simulink model "BLDCmotorControl_FOC_R2017b"  (R2017b)
settings: Solver=FixedStepDiscrete  StartTime=0  StopTime=1  FixedStep=Ts  MaxStep=1e-6  RelTol=1e-6  AbsTol=1e-6  EnableMultiTasking=on
PreLoadFcn:
  | addpath(genpath('01_Libraries'));
  | addpath(genpath('02_Figures'));
InitFcn:
  | init_model;
values from neighbouring files (symbols this model uses):
  a_elecAngle = 60    [init_model_Ffwd.m]
  a_elecPeriod = 360    [init_model_Ffwd.m]
  b_DCLinkCurrAvail = 0    [init_model_Ffwd.m]
  b_selPhaABCurrMeas = 1    [init_model_Ffwd.m]
  cf_speedCoef = round(f_ctrl * a_mechAngle * (pi/180) * (30/pi))    [init_model_Ffwd.m]
  i_thresOutlier = 200    [init_model_Ffwd.m]
  n_commAcvLo = 15    [init_model_Ffwd.m]
  n_commDeacvHi = 30    [init_model_Ffwd.m]
  r_sin_M1 = sin((a_elecAngle_XA + 30)*(pi/180))    [init_model_Ffwd.m]
  r_whl = 6.5 * 2.54 * 1e-2 / 2    (= 0.08255)    [init_model_Ffwd.m]
  res_elecAngle = 2    [init_model_Ffwd.m]
  Ts = 5e-6    (= 5e-06)    [init_model_Ffwd.m]    (also in pe_electric_engine_dyno_data.m = 1e-05)
  Ts_ctrl = 6e-5    (= 6e-05)    [init_model_Ffwd.m]
  vec_hallToPos = [0 2 0 1 4 3 5 0]    [init_model_Ffwd.m]
  z_commutMap_M1 = [-1 -1  0  1  1  0 ... (first row only)    [init_model_Ffwd.m]
  z_ctrlTypSel = 1    [init_model_Ffwd.m]
  z_maxCntRst = 2000    [init_model_Ffwd.m]
undefined symbols (not defined in the file or in its folder): a_phaAdv_M1, b_phaAdvEna, CTRL_COMM, DiscIntNeverNeededParam, Down, dz_counterHi, dz_counterLo, Kb_Id, Kb_Iq, Kb_n, Ki_Id, Ki_Iq, Ki_n, Kp_Id, Kp_Iq, Kp_n, n_motPhaAdvEna, r_commDCDeacv, sigbuilder_block, Up, V_circleLim_M1, V_max, V_min
libraries: pePwmGenerator x7, BLDC_controller_Lib x6, powerlib x6, simulink x5
(part 1 of 3)
Description:
  | This example illustrates use of the BLDC in a closed-loop
  | speed and voltage control on a 1 kW, 3000 rpm industrial motor
  | 
  | 
  | Copyright 2008-2019 The MathWorks, Inc.
settings Model: ExtModeAutoUpdateStatusClock=off  TunableVars=Ki_Id,Ki_Iq,Kp_Id,Kp_Iq,a_phaAdv_M1,b_phaAdvEna,cf_speedCoef,cf_speedFilt,dz_counterHi,dz_counterLo,f_ctrl,n_commAcvLo,n_commDeacvHi,n_motPhaAdvEna,r_commDCDeacv,r_phaAdvDC_XA,z_ctrlTypSel,z_maxCntRst  TunableVarsStorageClass=Auto,Auto,Auto,Auto,Auto,Auto,Auto,Auto,Auto,Auto,Auto,Auto,Auto,Auto,Auto,Auto,Auto,Auto  TunableVarsTypeQualifier=,,,,,,,,,,,,,,,,,  Creator=MathWorks  LastModifiedBy=37ef
settings SolverCC: AutoInsertRateTranBlk=on
settings DataIOCC: LimitDataPoints=on  SaveFormat=Array  ReturnWorkspaceOutputs=on  SignalLoggingName=sigsOut
settings OptimizationCC: DefaultParameterBehavior=Inlined  UseDivisionForNetSlopeComputation=on  UseFloatMulNetSlope=on  UseSpecifiedMinMax=on  InlineInvariantSignals=on  PassReuseOutputArgsAs=Individual arguments  ExpressionDepthLimit=2147483647  ZeroExternalMemoryAtStartup=off  ZeroInternalMemoryAtStartup=off  NoFixptDivByZeroProtection=on  EfficientFloat2IntCast=on  LifeSpan=1  OptimizeBlockOrder=speed  DifferentSizesBufferReuse=on
settings DebuggingCC: ReadBeforeWriteMsg=DisableAll  WriteAfterWriteMsg=DisableAll  WriteAfterReadMsg=DisableAll  UnderspecifiedInitializationDetection=Classic  InheritedTsInSrcMsg=none  MultiTaskDSMMsg=none  MultiTaskCondExecSysMsg=none  ParameterTunabilityLossMsg=error  FcnCallInpInsideContextMsg=warning  StateNameClashWarn=warning  SFUnexpectedBacktrackingDiag=warning  SFNoUnconditionalDefaultTransitionDiag=warning  SFExecutionAtInitializationDiag=none
settings HardwareCC: ProdBitPerPointer=32  ProdBitPerSizeT=32  ProdBitPerPtrDiffT=32  ProdLargestAtomicInteger=Long  ProdLargestAtomicFloat=Double  ProdWordSize=32  ProdHWDeviceType=ARM Compatible->ARM Cortex  TargetBitPerPointer=64  TargetBitPerSizeT=64  TargetBitPerPtrDiffT=64  TargetLongLongMode=on  TargetIntDivRoundTo=Zero  TargetEndianess=LittleEndian  TargetWordSize=64  TargetHWDeviceType=MATLAB Host  ProdEqTarget=off
settings ModelReferenceCC: UpdateModelReferenceTargets=IfOutOfDate  PropagateSignalLabelsOutOfModel=off
settings SFSimCC: SFSimEcho=off  MATLABDynamicMemAlloc=off
settings RTWCC: SystemTargetFile=ert.tlc  GenCodeOnly=on  TemplateMakefile=ert_default_tmf  GenerateReport=on  BuildConfiguration=Faster Runs  IncludeHyperlinkInReport=on  LaunchReport=on  GenerateTraceInfo=on  GenerateTraceReport=on  GenerateTraceReportSl=on  GenerateTraceReportSf=on  GenerateTraceReportEml=on  GenerateCodeMetricsReport=on  GenerateCodeReplacementReport=on
settings CodeAppCC: ForceParamTrailComments=on  IgnoreCustomStorageClasses=off  OperatorAnnotations=on  SimulinkDataObjDesc=on  SFDataObjDesc=on  CustomSymbolStrGlobalVar=rt$N$M  CustomSymbolStrType=$N$M  CustomSymbolStrFcn=$N$M$F  CustomSymbolStrMacro=$N$M  InsertBlockDesc=on
settings ERTTargetCC: GenerateSampleERTMain=on  IncludeMdlTerminateFcn=off  CombineSignalStateStructs=on  SuppressErrorStatus=on  MultiInstanceERTCode=on  CodeInterfacePackaging=Reusable function  SupportNonFinite=off  SupportComplex=off  InlinedParameterPlacement=NonHierarchical  RootIOFormat=Part of model data structure  ERTCustomFileTemplate=example_file_process.tlc  ERTFilePackagingFormat=CompactWithDataFile  PreserveStaticInFcnDecls=off
settings ConfigComp: CovMetricSettings=dw  CovHtmlReporting=on  CovSaveCumulativeToWorkspaceVar=on  CovSaveSingleToWorkspaceVar=on  CovExternalEMLEnable=off  CovSFcnEnable=off
settings SimscapeCC: SimscapeNormalizeSystem=off

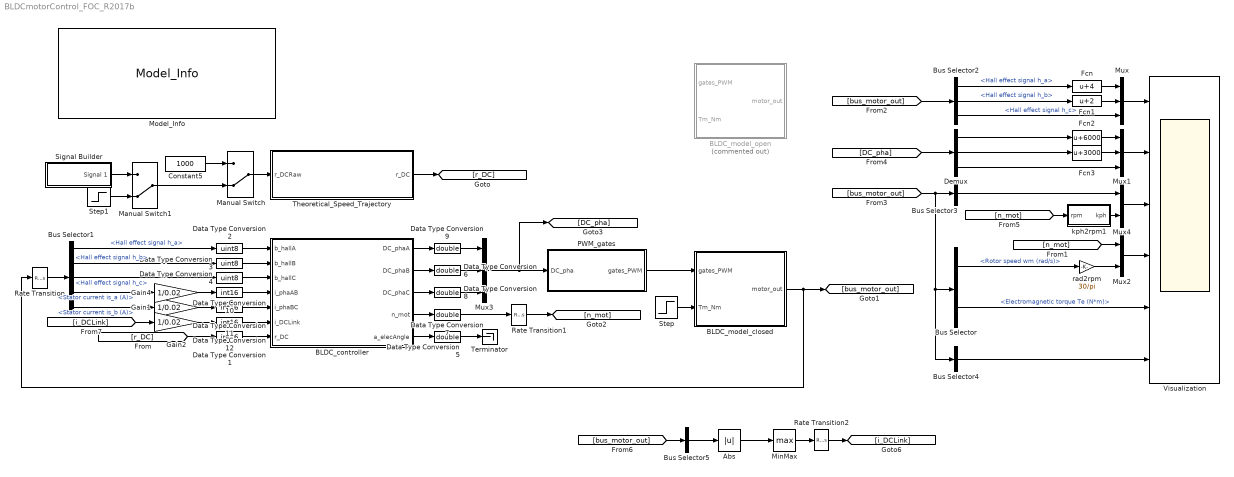
== system BLDCmotorControl_FOC_R2017b ==
  Abs : Abs
  BLDC_controller : Subsystem  TreatAsAtomicUnit=on  SystemSampleTime=Ts_ctrl
  BLDC_model_closed : Subsystem
      mask help: Simulink:masks:GenSFuncDesc_MD
      mask Help: eval('feval(''rtwprivate'',''rtwhelpview'',''rtw_sfcn_block'')');
  BLDC_model_open : Subsystem  Commented=on
  Bus Selector : BusSelector  OutputSignals=Rotor speed wm (rad/s),Electromagnetic torque Te (N*m)
  Bus Selector1 : BusSelector  OutputSignals=Hall effect signal h_a,Hall effect signal h_b,Hall effect signal h_c,Stator current is_a (A),Stator current is_b (A)
  Bus Selector2 : BusSelector  OutputSignals=Hall effect signal h_a,Hall effect signal h_b,Hall effect signal h_c
  Bus Selector3 : BusSelector  OutputSignals=Stator current is_a (A),Stator current is_b (A),Stator current is_c (A)  OutputAsBus=on
  Bus Selector4 : BusSelector  OutputSignals=Stator back EMF e_a (V),Stator back EMF e_b (V),Stator back EMF e_cV)  OutputAsBus=on
  Bus Selector5 : BusSelector  OutputSignals=Stator current is_a (A),Stator current is_b (A),Stator current is_c (A)  OutputAsBus=on
  Constant5 : Constant  Value=1000  OutDataTypeStr=double
  Data Type Conversion{1,10..12} (4 alike) : DataTypeConversion  OutDataTypeStr=int16  RndMeth=Zero
  Data Type Conversion2 : DataTypeConversion  OutDataTypeStr=uint8  RndMeth=Zero
  Data Type Conversion3 : DataTypeConversion  OutDataTypeStr=uint8  RndMeth=Zero
  Data Type Conversion4 : DataTypeConversion  OutDataTypeStr=uint8  RndMeth=Zero
  Data Type Conversion{5..9} (5 alike) : DataTypeConversion  OutDataTypeStr=double  RndMeth=Zero
  Demux : Demux  Outputs=3
  Fcn : Fcn  Expr=u+4
  Fcn1 : Fcn  Expr=u+2
  Fcn2 : Fcn  Expr=u+6000
  Fcn3 : Fcn  Expr=u+3000
  Gain1 : Gain  Tag=struct('comment',struct('text','','placement',1),'logdata',struct('maxnumvals',inf,'plotchannels',[],'loggingmode',3,'channels',1),'output',struct('variable','','description','','name','$S_$B','width',1,'address','','max',NaN,'min',NaN,'class','default','type','CONTINUOUS','scaling','','lsb',1,'offset',0,'arb',0,'freeze',1,'unit','','autoscalingmode',1,'lowerheadroom',1,'upperheadroom',1,'headroomunit','bit','keepdatatype',1,'checkmin',0,'checkmax',0,'castoutput',0,'show',0),'gain',struct('variable','','description','','name','$S_$B_gain','width',1,'address','','max',NaN,'min',NaN,'class','default','type','CONTINUOUS','scaling','','lsb',1,'offset',0,'arb',0,'freeze',1,'unit','','keepdatatype',1,'value','1','scalar',0,'tolerance',1),'scalingvalid',0,'date',730486)  Gain=1/0.02  RndMeth=Zero  SaturateOnIntegerOverflow=on  OutDataTypeStr=Inherit: Same as input  ParamDataTypeStr=Inherit: Same as input
  Gain2 : Gain  Tag=struct('comment',struct('text','','placement',1),'logdata',struct('maxnumvals',inf,'plotchannels',[],'loggingmode',3,'channels',1),'output',struct('variable','','description','','name','$S_$B','width',1,'address','','max',NaN,'min',NaN,'class','default','type','CONTINUOUS','scaling','','lsb',1,'offset',0,'arb',0,'freeze',1,'unit','','autoscalingmode',1,'lowerheadroom',1,'upperheadroom',1,'headroomunit','bit','keepdatatype',1,'checkmin',0,'checkmax',0,'castoutput',0,'show',0),'gain',struct('variable','','description','','name','$S_$B_gain','width',1,'address','','max',NaN,'min',NaN,'class','default','type','CONTINUOUS','scaling','','lsb',1,'offset',0,'arb',0,'freeze',1,'unit','','keepdatatype',1,'value','1','scalar',0,'tolerance',1),'scalingvalid',0,'date',730486)  Gain=1/0.02  RndMeth=Zero  SaturateOnIntegerOverflow=on  OutDataTypeStr=Inherit: Same as input  ParamDataTypeStr=Inherit: Same as input
  Gain4 : Gain  Tag=struct('comment',struct('text','','placement',1),'logdata',struct('maxnumvals',inf,'plotchannels',[],'loggingmode',3,'channels',1),'output',struct('variable','','description','','name','$S_$B','width',1,'address','','max',NaN,'min',NaN,'class','default','type','CONTINUOUS','scaling','','lsb',1,'offset',0,'arb',0,'freeze',1,'unit','','autoscalingmode',1,'lowerheadroom',1,'upperheadroom',1,'headroomunit','bit','keepdatatype',1,'checkmin',0,'checkmax',0,'castoutput',0,'show',0),'gain',struct('variable','','description','','name','$S_$B_gain','width',1,'address','','max',NaN,'min',NaN,'class','default','type','CONTINUOUS','scaling','','lsb',1,'offset',0,'arb',0,'freeze',1,'unit','','keepdatatype',1,'value','1','scalar',0,'tolerance',1),'scalingvalid',0,'date',730486)  Gain=1/0.02  RndMeth=Zero  SaturateOnIntegerOverflow=on  OutDataTypeStr=Inherit: Same as input  ParamDataTypeStr=Inherit: Same as input
  Manual Switch : ManualSwitch  CurrentSetting=0
  Manual Switch1 : ManualSwitch  CurrentSetting=0
  MinMax : MinMax  Function=max
  Model_Info : BLDC_controller_Lib/Model_Info
  Mux : Mux  Inputs=3
  Mux1 : Mux  Inputs=3
  Mux2 : Mux  Inputs=2
  Mux3 : Mux  Inputs=3
  Mux4 : Mux  Inputs=2
  PWM_gates : Subsystem
  Rate Transition : RateTransition  Integrity=off  Deterministic=off
  Rate Transition1 : RateTransition  Integrity=off  Deterministic=off
  Rate Transition2 : RateTransition  Integrity=off  Deterministic=off
  Signal Builder : Subsystem  Tag=STV Subsys  LoadFcn=sigbuilder_block('load');  StartFcn=sigbuilder_block('start');  StopFcn=sigbuilder_block('stop');  ClipboardFcn=sigbuilder_block('clipboard');  mask(Sigbuilder block){tuvar=[0:10]}
      mask help: Simulink:masks:SigbuilderBlock_MD
      mask init:
      | if ~strcmp(get_param(bdroot(gcbh),'SimulationStatus'),'stopped') tuvar = sigbuilder_block('maskInit'); end
      settings: CopyFcn=sigbuilder_block('copy');  DeleteFcn=sigbuilder_block('delete');  ModelCloseFcn=sigbuilder_block('modelClose');  PreSaveFcn=sigbuilder_block('preSave');  PauseFcn=sigbuilder_block('pause');  ContinueFcn=sigbuilder_block('continue');  NameChangeFcn=sigbuilder_block('namechange');  OpenFcn=sigbuilder_block('open',[141.283 165.057 550.868 400.075 ]);  CloseFcn=sigbuilder_block('close');
      mask Display: plot(0, 0, 100, 100,[2, 2, 32, 32, 2], [68, 8, 8, 68, 68],[32, 2], [38, 38], [32, 19, 2],[53, 60, 44], [32, 17, 17, 2],[16, 16, 31, 31]);txt = getActiveGroup(gcbh);text(2, 100, txt,'verticalAlignment', 'top');
  Step : Step  Time=0  After=0.5  SampleTime=0
  Step1 : Step  Time=0.25  Before=1000  After=-1000
  Terminator : Terminator
      settings: Tag=Controls_Lib  Description=Terminator  CopyFcn=Lib_CopyFcn(gcb);  PreDeleteFcn=Lib_PreDeleteFcn(gcb);
  Theoretical_Speed_Trajectory : Subsystem
  Visualization : Scope  NumInputPorts=6
  kph2rpm1 : Subsystem
  rad2rpm : Gain  Gain=30/pi
  wires:
  Mux2/1 -> Visualization/4
  Bus Selector/1 -> rad2rpm/1  "<Rotor speed wm (rad/s)>"
  Bus Selector/2 -> Visualization/5  "<Electromagnetic torque Te (N*m)>"
  Bus Selector2/3 -> Mux/3  "<Hall effect signal h_c>"
  Bus Selector2/2 -> Fcn1/1  "<Hall effect signal h_b>"
  Bus Selector2/1 -> Fcn/1  "<Hall effect signal h_a>"
  Fcn1/1 -> Mux/2
  Mux/1 -> Visualization/1
  Fcn/1 -> Mux/1
  Demux/1 -> Fcn2/1
  Demux/2 -> Fcn3/1
  Fcn2/1 -> Mux1/1
  Fcn3/1 -> Mux1/2
  Demux/3 -> Mux1/3
  Mux1/1 -> Visualization/2
  Bus Selector4/1 -> Visualization/6
  rad2rpm/1 -> Mux2/2
  BLDC_controller/4(n_mot) -> Data Type Conversion7/1
  BLDC_model_closed/1(motor_out) -> Rate Transition/1, [bus_motor_out]
  Step/1 -> BLDC_model_closed/2(Tm_Nm)
  Bus Selector1/2 -> Data Type Conversion3/1  "<Hall effect signal h_b>"
  Bus Selector1/1 -> Data Type Conversion2/1  "<Hall effect signal h_a>"
  Bus Selector1/3 -> Data Type Conversion4/1  "<Hall effect signal h_c>"
  Rate Transition/1 -> Bus Selector1/1
  Data Type Conversion2/1 -> BLDC_controller/1("b_hallA ")
  Data Type Conversion3/1 -> BLDC_controller/2(b_hallB)
  Data Type Conversion4/1 -> BLDC_controller/3(b_hallC)
  Theoretical_Speed_Trajectory/1(r_DC) -> [r_DC]
  [r_DC] -> Data Type Conversion1/1
  Data Type Conversion1/1 -> BLDC_controller/7(r_DC)
  BLDC_controller/2(DC_phaB) -> Data Type Conversion6/1
  BLDC_controller/3(DC_phaC) -> Data Type Conversion8/1
  BLDC_controller/1(DC_phaA) -> Data Type Conversion9/1
  Data Type Conversion7/1 -> Rate Transition1/1
  BLDC_controller/5(a_elecAngle) -> Data Type Conversion5/1
  Mux3/1 -> [DC_pha], PWM_gates/1(DC_pha)
  PWM_gates/1(gates_PWM) -> BLDC_model_closed/1(gates_PWM)
  Rate Transition1/1 -> [n_mot]
  [n_mot] -> Mux2/1
  [bus_motor_out] -> Bus Selector2/1
  [bus_motor_out] -> Bus Selector3/1, Bus Selector4/1, Bus Selector/1
  [DC_pha] -> Demux/1
  Manual Switch/1 -> Theoretical_Speed_Trajectory/1(r_DCRaw)
  Constant5/1 -> Manual Switch/1
  Signal Builder/1(Signal 1) -> Manual Switch1/1
  Manual Switch1/1 -> Manual Switch/2
  Step1/1 -> Manual Switch1/2
  Data Type Conversion5/1 -> Terminator/1
  Data Type Conversion8/1 -> Mux3/3
  Data Type Conversion6/1 -> Mux3/2
  Data Type Conversion9/1 -> Mux3/1
  [n_mot] -> kph2rpm1/1(rpm)
  Mux4/1 -> Visualization/3
  Bus Selector3/1 -> Mux4/1
  kph2rpm1/1(kph) -> Mux4/2
  Data Type Conversion10/1 -> BLDC_controller/4(i_phaAB)
  Data Type Conversion11/1 -> BLDC_controller/5(i_phaBC)
  Gain4/1 -> Data Type Conversion10/1
  Gain1/1 -> Data Type Conversion11/1
  [bus_motor_out] -> Bus Selector5/1
  Abs/1 -> MinMax/1
  Bus Selector5/1 -> Abs/1
  Data Type Conversion12/1 -> BLDC_controller/6(i_DCLink)
  Gain2/1 -> Data Type Conversion12/1
  [i_DCLink] -> Gain2/1
  MinMax/1 -> Rate Transition2/1
  Rate Transition2/1 -> [i_DCLink]
  Bus Selector1/4 -> Gain4/1  "<Stator current is_a (A)>"
  Bus Selector1/5 -> Gain1/1  "<Stator current is_b (A)>"

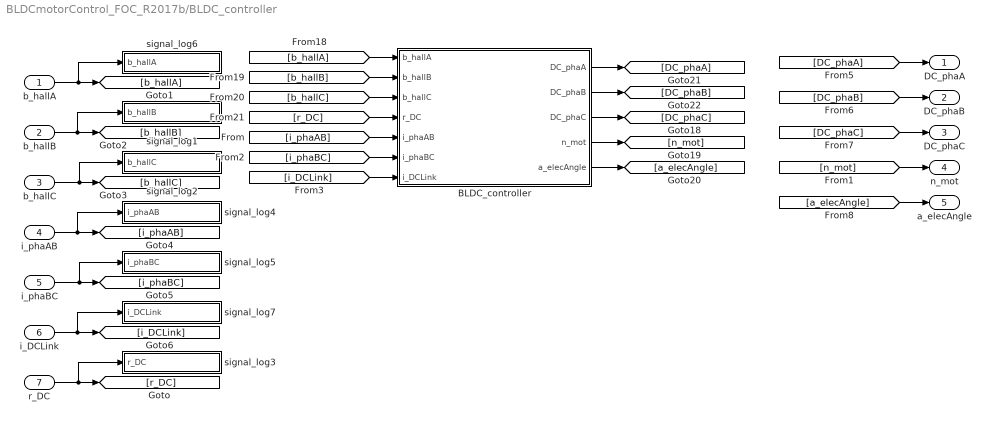
== system BLDCmotorControl_FOC_R2017b/BLDC_controller ==
  "b_hallA " : Inport
  b_hallB : Inport  Port=2
  b_hallC : Inport  Port=3
  i_phaAB : Inport  Port=4
  i_phaBC : Inport  Port=5
  i_DCLink : Inport  Port=6
  r_DC : Inport  Port=7
  BLDC_controller : Subsystem  SystemSampleTime=1e-5
  signal_log1 : Subsystem
  signal_log2 : Subsystem
  signal_log3 : Subsystem
  signal_log4 : Subsystem
  signal_log5 : Subsystem
  signal_log6 : Subsystem
  signal_log7 : Subsystem
  DC_phaA : Outport
  DC_phaB : Outport  Port=2
  DC_phaC : Outport  Port=3
  n_mot : Outport  Port=4
  a_elecAngle : Outport  Port=5
  wires:
  "b_hallA "/1 -> signal_log6/1(b_hallA), [b_hallA]
  b_hallB/1 -> signal_log1/1(b_hallB), [b_hallB]
  b_hallC/1 -> signal_log2/1(b_hallC), [b_hallC]
  [n_mot] -> n_mot/1
  [DC_phaA] -> DC_phaA/1
  [DC_phaB] -> DC_phaB/1
  [DC_phaC] -> DC_phaC/1
  r_DC/1 -> signal_log3/1(r_DC), [r_DC]
  [a_elecAngle] -> a_elecAngle/1
  [r_DC] -> BLDC_controller/4(r_DC)
  [b_hallC] -> BLDC_controller/3(b_hallC)
  [b_hallB] -> BLDC_controller/2(b_hallB)
  [b_hallA] -> BLDC_controller/1("b_hallA ")
  BLDC_controller/5(a_elecAngle) -> [a_elecAngle]
  BLDC_controller/4(n_mot) -> [n_mot]
  BLDC_controller/3(DC_phaC) -> [DC_phaC]
  BLDC_controller/2(DC_phaB) -> [DC_phaB]
  BLDC_controller/1(DC_phaA) -> [DC_phaA]
  i_phaBC/1 -> [i_phaBC], signal_log5/1(i_phaBC)
  i_phaAB/1 -> [i_phaAB], signal_log4/1(i_phaAB)
  [i_phaAB] -> BLDC_controller/5(i_phaAB)
  [i_phaBC] -> BLDC_controller/6(i_phaBC)
  i_DCLink/1 -> signal_log7/1(i_DCLink), [i_DCLink]
  [i_DCLink] -> BLDC_controller/7(i_DCLink)

== system BLDCmotorControl_FOC_R2017b/BLDC_model_closed ==
  gates_PWM : Inport
  Tm_Nm : Inport  Port=2
  BLDC_model_sfcn : S-Function  FunctionName=BLDC_model_sf  SFunctionModules=""  SFunctionDeploymentMode=off  EnableBusSupport=off  SFcnStateName=DWORK0  mask{rtw_sf_name=BLDC_model_sf, showVar=off}
      mask prompts: rtw_sf_name "Simulink:masks:GenSFuncName_MP"; showVar "Simulink:masks:GenSFuncShowModuleList_MP"
      mask help: Simulink:masks:GenSFuncDesc_MD
      mask init:
      | displist = '';
      | if ~strcmp(get_param(gcb, 'FunctionName'), rtw_sf_name);
      |   set_param(gcb, 'FunctionName', rtw_sf_name);
      | end
      | % Check if we are generating code
      | rtw_mode = false;
      | if strcmpi(get_param(bdroot(gcb),'SimulationStatus'),'Initializing')
      | 	rtw_mode = strcmpi(get_param(bdroot(gcb),'BuildingRTWCode'),'on') && ...
      | 		~strcmpi(get_param(bdroot(gcb),'TargetStyle'),'SimulationTarget');
      | end
      | if showVar || rtw_mode
      | 	if exist('rtwsfunc') == 2 | exist('rtwsfunc') == 6
      | 		tmplist = rtwsfunc(rtw_sf_name,gcb);
      | 		tmplist = DAStudio.message('Simulink:masks:GenSFuncListOfModules_IC', tmplist);
      | 	elseif showVar
      | 		tmplist1 = DAStudio.message('Simulink:masks:GenSFuncListOfModules_IC', '');
      |         tmplist2 = DAStudio.message('Simulink:masks:GenSFuncNotLicensed_IC');
      |         tmplist = [tmplist1 tmplist2];
      |  	end
      | end
      | if showVar
      |   displist = tmplist;
      | end
      settings: SFcnIsStateOwnerBlock=on
      settings: CopyFcn=|
      | if ~strcmp(get_param(gcb,'Linkstatus'),'none') && ...
      | ~strcmp(get_param(gcb,'Linkstatus'),'implicit')
      |   set_param(gcb,'LinkStatus','none');
      | end
      mask Help: eval('feval(''rtwprivate'',''rtwhelpview'',''rtw_sfcn_block'')');
      mask Display:
      | port_label('input',1,'gates_PWM');
      | port_label('input',2,'Tm_Nm');
      | port_label('output',1,'Stator current is_a (A)');
      | port_label('output',2,'Stator current is_b (A)');
      | port_label('output',3,'Stator current is_c (A)');
      | port_label('output',4,'Stator back EMF e_a (V)');
      | port_label('output',5,'Stator back EMF e_b (V)');
      | port_label('output',6,'Stator back EMF e_cV)');
      | port_label('output',7,'Hall effect signal h_a');
      | port_label('output',8,'Hall effect signal h_b');
      | port_label('output',9,'Hall effect signal h_c');
      | port_label('output',10,'Rotor speed wm (rad/s)');
      | port_label('output',11,'Rotor angle thetam (rad)');
      | port_label('output',12,'Electromagnetic torque Te (N*m)');
  __InputSSForSFun__ : Subsystem
  __OutputSSForSFun__ : Subsystem
  motor_out : Outport
  wires:
  gates_PWM/1 -> __InputSSForSFun__/1(gates_PWM)
  Tm_Nm/1 -> __InputSSForSFun__/2(Tm_Nm)
  __InputSSForSFun__/1(__UniqueOutportName__1__) -> BLDC_model_sfcn/1
  __InputSSForSFun__/2(__UniqueOutportName__2__) -> BLDC_model_sfcn/2
  BLDC_model_sfcn/1 -> __OutputSSForSFun__/1(__UniqueInportName__1__)
  BLDC_model_sfcn/2 -> __OutputSSForSFun__/2(__UniqueInportName__2__)
  BLDC_model_sfcn/3 -> __OutputSSForSFun__/3(__UniqueInportName__3__)
  BLDC_model_sfcn/4 -> __OutputSSForSFun__/4(__UniqueInportName__4__)
  BLDC_model_sfcn/5 -> __OutputSSForSFun__/5(__UniqueInportName__5__)
  BLDC_model_sfcn/6 -> __OutputSSForSFun__/6(__UniqueInportName__6__)
  BLDC_model_sfcn/7 -> __OutputSSForSFun__/7(__UniqueInportName__7__)
  BLDC_model_sfcn/8 -> __OutputSSForSFun__/8(__UniqueInportName__8__)
  BLDC_model_sfcn/9 -> __OutputSSForSFun__/9(__UniqueInportName__9__)
  BLDC_model_sfcn/10 -> __OutputSSForSFun__/10(__UniqueInportName__10__)
  BLDC_model_sfcn/11 -> __OutputSSForSFun__/11(__UniqueInportName__11__)
  BLDC_model_sfcn/12 -> __OutputSSForSFun__/12(__UniqueInportName__12__)
  __OutputSSForSFun__/1(motor_out) -> motor_out/1

== system BLDCmotorControl_FOC_R2017b/BLDC_model_open ==
  gates_PWM : Inport
  Tm_Nm : Inport  Port=2
  Constant1 : Constant  Value=36
  Controlled Voltage Source1 : powerlib/Electrical Sources/Controlled Voltage Source  Initialize=on  Source_Type=DC  Amplitude=500  Phase=0  Frequency=0  Measurements=None
  Current Measurement : powerlib/Measurements/Current Measurement  PhasorSimulation=off  OutputType=Magnitude  PSBequivalent=0
  Permanent Magnet Synchronous Machine : powerlib/Machines/Permanent Magnet Synchronous Machine  NbPhases=3  FluxDistribution=Trapezoidal  RotorType=Round  MechanicalLoad=Torque Tm  PresetModel=No  ShowDetailedParameters=on  MeasurementBus=off  Resistance=0.18  Inductance=0.000835  dqInductances=[8.5e-3, 8.5e-3]  La=0.000835  MachineConstant=Flux linkage established by magnets (V.s)  Flux=0.0142879  VoltageCst=44.8868  TorqueCst=0.42864  Flat=120  Mechanical=[0.00621417 0.000303448 15]  PolePairs=15  InitialConditions=[0,0, 0,0]  InitialConditions5ph=[0 0 0 0 0 0]  TsPowergui=0  TsBlock=-1  RefAngle=90 degrees behind phase A axis (modified Park)
      settings: SourceProductName=Simscape Power Systems
  Universal Bridge1 : powerlib/Power Electronics/Universal Bridge  Arms=3  SnubberResistance=5000  SnubberCapacitance=inf  Device=MOSFET / Diodes  Ron=1e-3  Lon=0  ForwardVoltages="[  0  0  ]"  ForwardVoltage=0  GTOparameters=[ 10e-6 , 20e-6 ]  IGBTparameters=[ 1e-6 , 2e-6 ]  Measurements=None  Measurements_2=None  converterType=Rectifier
  Vab : Scope
  Voltage Measurement : powerlib/Measurements/Voltage Measurement  PhasorSimulation=off  OutputType=Complex  PSBequivalent=0
  iDC : Scope
  powergui : powerlib/powergui  Priority=2  SimulationMode=Discrete  SampleTime=Ts  frequency=60  Iterations=50  frequencyindice=0  Pbase=100e6  ErrMax=1e-4  UnitsV=kV  UnitsW=MW  buscounter=0  FunctionMessages=off  echomessages=off  EnableUseOfTLC=off  CurrentSourceSwitches=off  DisableSnubberDevices=off  DisableRonSwitches=off  DisableVfSwitches=off  DisplayEquations=off  SolverType=Tustin/Backward Euler (TBE)  Interpol=off  ExternalGateDelay=off  methode=off  Ts=0  x0status=blocks  SPID=off  SwTol=0  HookPort=off  RestoreLinks=warning  ResistiveCurrentMeasurement=off  Frange=[0:2:500]  Ylog=off  Xlog=on  ShowGrid=off  save=off  variable=ZData  structure=0  ZoomFFT=on  StartTime=0.0  cycles=1  DisplayStyle=1  fundamental=60  FreqAxis=off  MaxFrequency=1000  frequencyindicesteady=1  RmsSteady=1  display=off
  signal_log6 : Subsystem
  motor_out : Outport
  wires:
  Constant1/1 -> Controlled Voltage Source1/1
  Tm_Nm/1 -> Permanent Magnet Synchronous Machine/1
  gates_PWM/1 -> Universal Bridge1/1
  Permanent Magnet Synchronous Machine/1 -> motor_out/1
  Voltage Measurement/1 -> Vab/1
  Current Measurement/1 -> iDC/1, signal_log6/1(i_DC)
  connections:
  Voltage Measurement/LConn2 -- Permanent Magnet Synchronous Machine/LConn2 -- Universal Bridge1/LConn2
  Universal Bridge1/LConn3 -- Permanent Magnet Synchronous Machine/LConn3
  Universal Bridge1/LConn1 -- Permanent Magnet Synchronous Machine/LConn1 -- Voltage Measurement/LConn1
  Current Measurement/RConn1 -- Controlled Voltage Source1/LConn1
  Current Measurement/LConn1 -- Universal Bridge1/RConn2
  Controlled Voltage Source1/RConn1 -- Universal Bridge1/RConn1

== system BLDCmotorControl_FOC_R2017b/PWM_gates ==
  DC_pha : Inport
  Abs : Abs  OutDataTypeStr=Inherit: Inherit via back propagation  RndMeth=Zero
  Abs1 : Abs  OutDataTypeStr=Inherit: Inherit via back propagation  RndMeth=Zero
  Abs2 : Abs  OutDataTypeStr=Inherit: Inherit via back propagation  RndMeth=Zero
  Constant4 : Constant  Value=0  OutDataTypeStr=Inherit: Inherit via back propagation
  Demux : Demux  Outputs=3
  Gain8 : Gain  Gain=1/1000  OutDataTypeStr=Inherit: Inherit via back propagation  RndMeth=Zero
  MinMax : MinMax  Inputs=2  OutDataTypeStr=Inherit: Inherit via back propagation  RndMeth=Zero
  MinMax1 : MinMax  Function=max  Inputs=2  OutDataTypeStr=Inherit: Inherit via back propagation  RndMeth=Zero
  MinMax2 : MinMax  Inputs=2  OutDataTypeStr=Inherit: Inherit via back propagation  RndMeth=Zero
  MinMax3 : MinMax  Function=max  Inputs=2  OutDataTypeStr=Inherit: Inherit via back propagation  RndMeth=Zero
  MinMax4 : MinMax  Inputs=2  OutDataTypeStr=Inherit: Inherit via back propagation  RndMeth=Zero
  MinMax5 : MinMax  Function=max  Inputs=2  OutDataTypeStr=Inherit: Inherit via back propagation  RndMeth=Zero
  Mux4 : Mux  Inputs=6
  PWM_generator{,7..11} (6 alike) : pePwmGenerator/PWM Generator  Commented=on  CarrCount=Up-Down  Tper=5e-5  Ts=5e-6
      settings: SourceProductName=The database C:\Users\37ef\AppData\Roaming\MathWorks\MATLAB\R2017b\slblocks_master.db is locked, or a table in the database is locked. (database is locked)
  PWM_generator1 : Subsystem
      mask help: Simulink:masks:GenSFuncDesc_MD
      mask Help: eval('feval(''rtwprivate'',''rtwhelpview'',''rtw_sfcn_block'')');
  PWM_generator12 : Subsystem
      mask help: Simulink:masks:GenSFuncDesc_MD
      mask Help: eval('feval(''rtwprivate'',''rtwhelpview'',''rtw_sfcn_block'')');
  PWM_generator2 : Subsystem
      mask help: Simulink:masks:GenSFuncDesc_MD
      mask Help: eval('feval(''rtwprivate'',''rtwhelpview'',''rtw_sfcn_block'')');
  PWM_generator3 : Subsystem
      mask help: Simulink:masks:GenSFuncDesc_MD
      mask Help: eval('feval(''rtwprivate'',''rtwhelpview'',''rtw_sfcn_block'')');
  PWM_generator4 : Subsystem
      mask help: Simulink:masks:GenSFuncDesc_MD
      mask Help: eval('feval(''rtwprivate'',''rtwhelpview'',''rtw_sfcn_block'')');
  PWM_generator5 : Subsystem
      mask help: Simulink:masks:GenSFuncDesc_MD
      mask Help: eval('feval(''rtwprivate'',''rtwhelpview'',''rtw_sfcn_block'')');
  PWM_generator6 : pePwmGenerator/PWM Generator  Commented=on  CarrCount=Up  Tper=5e-5  Ts=5e-6
      settings: SourceProductName=The database C:\Users\37ef\AppData\Roaming\MathWorks\MATLAB\R2017b\slblocks_master.db is locked, or a table in the database is locked. (database is locked)
  signal_log6 : Subsystem
  gates_PWM : Outport
  wires:
  PWM_generator4/1(PWM) -> Mux4/5
  Abs/1 -> PWM_generator1/1(DC)
  PWM_generator12/1(PWM) -> Mux4/1
  PWM_generator5/1(PWM) -> Mux4/6
  MinMax1/1 -> PWM_generator12/1(DC)
  PWM_generator3/1(PWM) -> Mux4/4
  PWM_generator1/1(PWM) -> Mux4/2
  MinMax5/1 -> PWM_generator4/1(DC)
  PWM_generator2/1(PWM) -> Mux4/3
  Abs2/1 -> PWM_generator5/1(DC)
  MinMax3/1 -> PWM_generator2/1(DC)
  Abs1/1 -> PWM_generator3/1(DC)
  Demux/1 -> MinMax/2, MinMax1/2
  MinMax4/1 -> Abs2/1
  Constant4/1 -> MinMax1/1, MinMax4/1, MinMax5/1, MinMax2/1, MinMax3/1, MinMax/1
  MinMax2/1 -> Abs1/1
  Demux/2 -> MinMax2/2, MinMax3/2
  MinMax/1 -> Abs/1
  Demux/3 -> MinMax5/2, MinMax4/2
  Gain8/1 -> Demux/1
  Mux4/1 -> signal_log6/1(PWM), gates_PWM/1
  DC_pha/1 -> Gain8/1

== system BLDCmotorControl_FOC_R2017b/Signal Builder ==
  Demux : Demux  Tag=STV Demux  Outputs=1
  FromWs : FromWorkspace  Tag=STV FromWs  VariableName=tuvar
      SigBuilderData=|
      | common.afterFinalStr = 'Extrapolate'
      | common.sampleTime = '-1'
      | dataSet.timeRange = [0 1.5]
      | dataSet.name = 'Group 1'
      | sbobj.Groups.Name = 'Group 1'
      | sbobj.Groups.Signals.Name = 'Signal 1'
      | sbobj.Groups.Signals.XData = [0 0.2 0.4 0.6 0.8 1.5]
      | sbobj.Groups.Signals.YData = [0 800 800 600 -800 -800]
      | sbobj.Groups.TimeRange = [0 1.5]
  Signal 1 : Outport  Tag=STV Outport
  wires:
  Demux/1 -> Signal 1/1
  FromWs/1 -> Demux/1

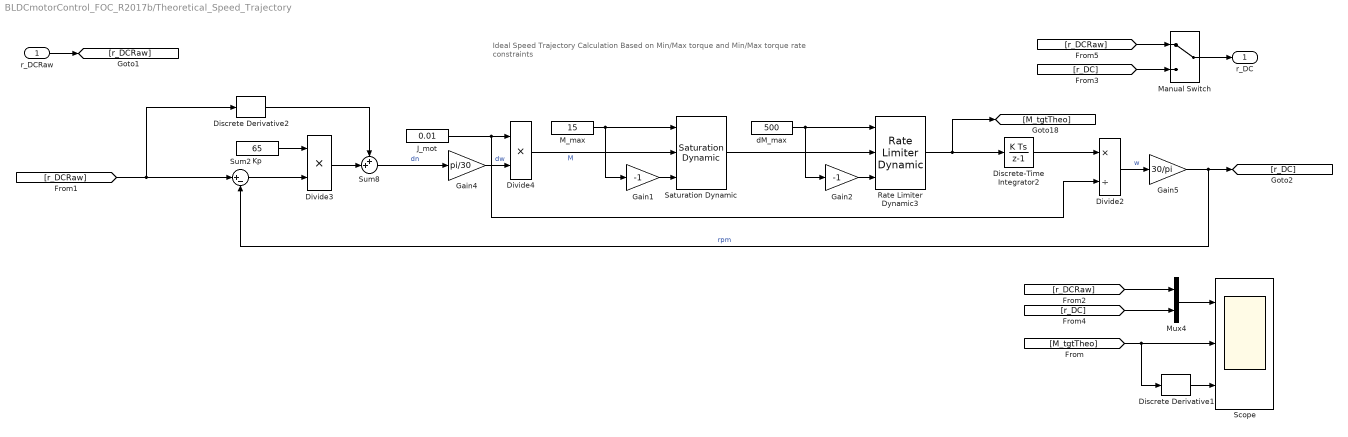
== system BLDCmotorControl_FOC_R2017b/Theoretical_Speed_Trajectory ==
  note: Ideal Speed Trajectory Calculation
      | Based on Min/Max torque and Min/Max torque rate constraints
  r_DCRaw : Inport
  Discrete Derivative1 : simulink/Discrete/Discrete Derivative  gainval=1.0  ICPrevScaledInput=0.0  OutMin=[]  OutMax=[]  OutDataType=fixdt(1, 16)  OutScaling=2^-10  DoSatur=off
  Discrete Derivative2 : simulink/Discrete/Discrete Derivative  gainval=1.0  ICPrevScaledInput=0.0  OutMin=[]  OutMax=[]  OutDataType=fixdt(1, 16)  OutScaling=2^-10  DoSatur=off
  Discrete-Time Integrator2 : DiscreteIntegrator  SampleTime=-1  ICPrevOutput=DiscIntNeverNeededParam  ICPrevScaledInput=DiscIntNeverNeededParam
  Divide2 : Product  Inputs=*/
  Divide3 : Product  Inputs=**
  Divide4 : Product  Inputs=**
  Gain1 : Gain  Gain=-1
  Gain2 : Gain  Gain=-1
  Gain4 : Gain  Gain=pi/30
  Gain5 : Gain  Gain=30/pi
  J_mot : Constant  Value=0.01  OutDataTypeStr=Inherit: Inherit via back propagation
  Kp : Constant  Value=65  OutDataTypeStr=Inherit: Inherit via back propagation
  M_max : Constant  Value=15  OutDataTypeStr=Inherit: Inherit via back propagation
  Manual Switch : ManualSwitch
  Mux4 : Mux  Inputs=2
  Rate Limiter Dynamic3 : simulink/Discontinuities/Rate Limiter Dynamic
      settings: SourceProductName=Simulink
  Saturation Dynamic : simulink/Discontinuities/Saturation Dynamic  OutMin=[]  OutMax=[]  OutDataTypeStr=Inherit: Same as second input  OutDataType=fixdt(1, 16)  OutScaling=2^-10  DoSatur=off
  Scope : Scope  NumInputPorts=3
  Sum2 : Sum  Inputs=|+-  RndMeth=Zero  OutDataTypeStr=Inherit: Same as first input
  Sum8 : Sum  Inputs=++|  RndMeth=Zero  OutDataTypeStr=Inherit: Same as first input
  dM_max : Constant  Value=500  OutDataTypeStr=Inherit: Inherit via back propagation
  r_DC : Outport
  wires:
  Gain4/1 -> Divide4/2  "dw"
  M_max/1 -> Gain1/1, Saturation Dynamic/1
  J_mot/1 -> Divide2/2, Divide4/1
  Divide2/1 -> Gain5/1  "w"
  [r_DCRaw] -> Discrete Derivative2/1, Sum2/1
  Divide4/1 -> Saturation Dynamic/2  "M"
  Gain1/1 -> Saturation Dynamic/3
  dM_max/1 -> Gain2/1, Rate Limiter Dynamic3/1
  Sum2/1 -> Divide3/2
  Divide3/1 -> Sum8/2
  Rate Limiter Dynamic3/1 -> [M_tgtTheo], Discrete-Time Integrator2/1
  Gain2/1 -> Rate Limiter Dynamic3/3
  Sum8/1 -> Gain4/1  "dn"
  Saturation Dynamic/1 -> Rate Limiter Dynamic3/2
  Gain5/1 -> [r_DC], Sum2/2  "rpm"
  Kp/1 -> Divide3/1
  Discrete-Time Integrator2/1 -> Divide2/1
  Mux4/1 -> Scope/1
  Discrete Derivative1/1 -> Scope/3
  Discrete Derivative2/1 -> Sum8/1
  [M_tgtTheo] -> Discrete Derivative1/1, Scope/2
  r_DCRaw/1 -> [r_DCRaw]
  [r_DCRaw] -> Mux4/1
  [r_DC] -> Mux4/2
  [r_DC] -> Manual Switch/2
  Manual Switch/1 -> r_DC/1
  [r_DCRaw] -> Manual Switch/1

== system BLDCmotorControl_FOC_R2017b/kph2rpm1 ==
  rpm : Inport
  Divide2 : Product  Inputs=**  RndMeth=Zero  OutDataTypeStr=Inherit: Same as first input
  Gain4 : Gain  Gain=pi/30  RndMeth=Zero  OutDataTypeStr=Inherit: Same as input
  Gain5 : Gain  Gain=3.6  RndMeth=Zero  OutDataTypeStr=Inherit: Same as input
  const2 : Constant  Value=r_whl  OutDataTypeStr=Inherit: Inherit via back propagation
  kph : Outport
  wires:
  rpm/1 -> Gain4/1
  Gain4/1 -> Divide2/1  "radps"
  const2/1 -> Divide2/2
  Divide2/1 -> Gain5/1  "mps"
  Gain5/1 -> kph/1

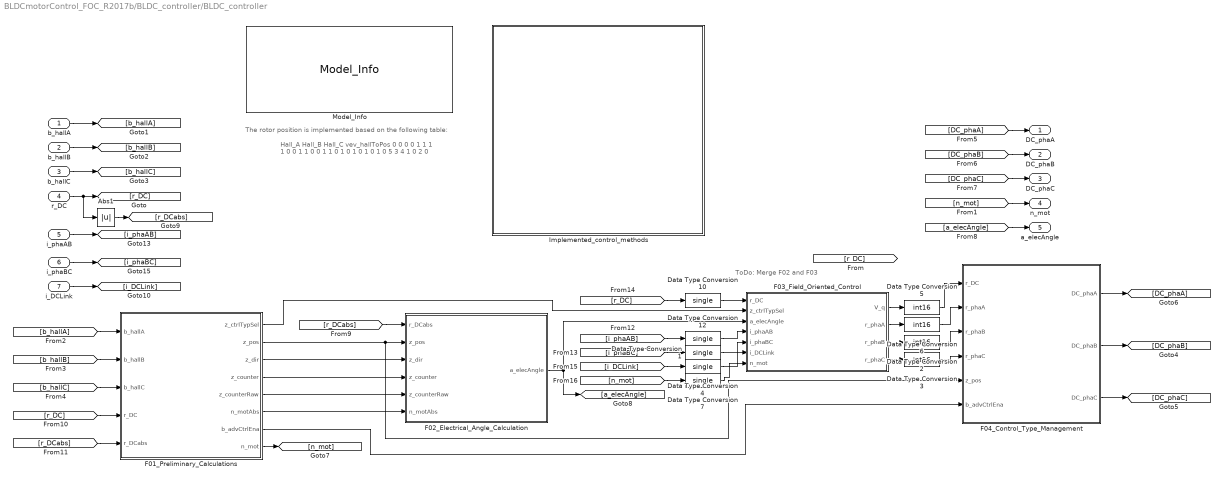
== system BLDCmotorControl_FOC_R2017b/BLDC_controller/BLDC_controller ==
  note: ToDo: Merge F02 and F03
  note: The rotor position is implemented based on the following table:
  note: Hall_A
      | Hall_B
      | Hall_C
      | vev_hallToPos
      |
      | 0
      | 0
      | 0
      | 0
      | 1
      | 1
      | 1
      | 1
      | 0
      | 0
      | 1
      | 1
      | 0
      | 0
      | 1
      | 1
      | 0
      | 1
      | 0
      | 1
      | 0
      | 1
      | 0
      | 1
      | 0
      | 5
      | 3
      | 4
      | 1
      | 0
      | 2
      | 0
  "b_hallA " : Inport
  b_hallB : Inport  Port=2
  b_hallC : Inport  Port=3
  r_DC : Inport  Port=4
  i_phaAB : Inport  Port=5
  i_phaBC : Inport  Port=6
  i_DCLink : Inport  Port=7
  Abs1 : Abs  OutDataTypeStr=Inherit: Inherit via back propagation  RndMeth=Zero
  Data Type Conversion{1,4,7,10,12} (5 alike) : DataTypeConversion  OutDataTypeStr=single
  Data Type Conversion{2..3,5..6} (4 alike) : DataTypeConversion  OutDataTypeStr=int16
  F01_Preliminary_Calculations : Subsystem
  F02_Electrical_Angle_Calculation : Subsystem
  F03_Field_Oriented_Control : Subsystem
  F04_Control_Type_Management : Subsystem
  Implemented_control_methods : Subsystem
      mask Display: image('control_methods.png')
  Model_Info : BLDC_controller_Lib/Model_Info
  DC_phaA : Outport
  DC_phaB : Outport  Port=2
  DC_phaC : Outport  Port=3
  n_mot : Outport  Port=4
  a_elecAngle : Outport  Port=5
  wires:
  "b_hallA "/1 -> [b_hallA]
  b_hallB/1 -> [b_hallB]
  b_hallC/1 -> [b_hallC]
  [n_mot] -> n_mot/1
  [DC_phaA] -> DC_phaA/1
  [b_hallA] -> F01_Preliminary_Calculations/1(b_hallA)
  [b_hallC] -> F01_Preliminary_Calculations/3(b_hallC)
  [b_hallB] -> F01_Preliminary_Calculations/2(b_hallB)
  F01_Preliminary_Calculations/2(z_pos) -> F04_Control_Type_Management/5(z_pos), F02_Electrical_Angle_Calculation/2(z_pos)
  F01_Preliminary_Calculations/3(z_dir) -> F02_Electrical_Angle_Calculation/3(z_dir)
  F01_Preliminary_Calculations/8("n_mot ") -> [n_mot]
  F01_Preliminary_Calculations/1(z_ctrlTypSel) -> F03_Field_Oriented_Control/2(z_ctrlTypSel)
  F02_Electrical_Angle_Calculation/1(a_elecAngle) -> [a_elecAngle], F03_Field_Oriented_Control/3(a_elecAngle)
  F03_Field_Oriented_Control/2(r_phaA) -> Data Type Conversion6/1
  F03_Field_Oriented_Control/3(r_phaB) -> Data Type Conversion2/1
  F03_Field_Oriented_Control/4("r_phaC ") -> Data Type Conversion3/1
  F04_Control_Type_Management/1(DC_phaA) -> [DC_phaA]
  F04_Control_Type_Management/2(DC_phaB) -> [DC_phaB]
  F04_Control_Type_Management/3("DC_phaC ") -> [DC_phaC]
  [DC_phaB] -> DC_phaB/1
  [DC_phaC] -> DC_phaC/1
  r_DC/1 -> [r_DC], Abs1/1
  [a_elecAngle] -> a_elecAngle/1
  [r_DCabs] -> F02_Electrical_Angle_Calculation/1(r_DCabs)
  [r_DC] -> F01_Preliminary_Calculations/4(r_DC)
  F01_Preliminary_Calculations/7(b_advCtrlEna) -> F04_Control_Type_Management/6(b_advCtrlEna)
  F01_Preliminary_Calculations/4(z_counter) -> F02_Electrical_Angle_Calculation/4(z_counter)
  F01_Preliminary_Calculations/5(z_counterRaw) -> F02_Electrical_Angle_Calculation/5(z_counterRaw)
  Abs1/1 -> [r_DCabs]
  [r_DCabs] -> F01_Preliminary_Calculations/5(r_DCabs)
  F01_Preliminary_Calculations/6(n_motAbs) -> F02_Electrical_Angle_Calculation/6(n_motAbs)
  [i_phaAB] -> Data Type Conversion12/1
  [i_phaBC] -> Data Type Conversion1/1
  [r_DC] -> Data Type Conversion10/1
  Data Type Conversion10/1 -> F03_Field_Oriented_Control/1(r_DC)
  Data Type Conversion6/1 -> F04_Control_Type_Management/2(r_phaA)
  Data Type Conversion2/1 -> F04_Control_Type_Management/3(r_phaB)
  Data Type Conversion3/1 -> F04_Control_Type_Management/4(r_phaC)
  Data Type Conversion12/1 -> F03_Field_Oriented_Control/4(i_phaAB)
  Data Type Conversion1/1 -> F03_Field_Oriented_Control/5(i_phaBC)
  i_phaAB/1 -> [i_phaAB]
  i_phaBC/1 -> [i_phaBC]
  i_DCLink/1 -> [i_DCLink]
  [i_DCLink] -> Data Type Conversion4/1
  Data Type Conversion4/1 -> F03_Field_Oriented_Control/6(i_DCLink)
  F03_Field_Oriented_Control/1(V_q) -> Data Type Conversion5/1
  Data Type Conversion5/1 -> F04_Control_Type_Management/1(r_DC)
  [n_mot] -> Data Type Conversion7/1
  Data Type Conversion7/1 -> F03_Field_Oriented_Control/7(n_mot)

== system BLDCmotorControl_FOC_R2017b/BLDC_controller/signal_log1 ==
  b_hallB : Inport
  Terminator_1 : Terminator
  wires:
  b_hallB/1 -> Terminator_1/1  "b_hallB"

== system BLDCmotorControl_FOC_R2017b/BLDC_controller/signal_log2 ==
  b_hallC : Inport
  Terminator_1 : Terminator
  wires:
  b_hallC/1 -> Terminator_1/1  "b_hallC"

== system BLDCmotorControl_FOC_R2017b/BLDC_controller/signal_log3 ==
  r_DC : Inport
  Terminator_1 : Terminator
  wires:
  r_DC/1 -> Terminator_1/1  "r_DC"

== system BLDCmotorControl_FOC_R2017b/BLDC_controller/signal_log4 ==
  i_phaAB : Inport
  Terminator_1 : Terminator
  wires:
  i_phaAB/1 -> Terminator_1/1  "i_phaAB"

== system BLDCmotorControl_FOC_R2017b/BLDC_controller/signal_log5 ==
  i_phaBC : Inport
  Terminator_1 : Terminator
  wires:
  i_phaBC/1 -> Terminator_1/1  "i_phaBC"

== system BLDCmotorControl_FOC_R2017b/BLDC_controller/signal_log6 ==
  b_hallA : Inport
  Terminator_1 : Terminator
  wires:
  b_hallA/1 -> Terminator_1/1  "b_hallA"

== system BLDCmotorControl_FOC_R2017b/BLDC_controller/signal_log7 ==
  i_DCLink : Inport
  Terminator_1 : Terminator
  wires:
  i_DCLink/1 -> Terminator_1/1  "i_DCLink"

== system BLDCmotorControl_FOC_R2017b/BLDC_model_closed/__InputSSForSFun__ ==
  gates_PWM : Inport
  Tm_Nm : Inport  Port=2
  __UniqueOutportName__1__ : Outport
  __UniqueOutportName__2__ : Outport  Port=2
  wires:
  gates_PWM/1 -> __UniqueOutportName__1__/1
  Tm_Nm/1 -> __UniqueOutportName__2__/1

== system BLDCmotorControl_FOC_R2017b/BLDC_model_closed/__OutputSSForSFun__ ==
  __UniqueInportName__1__ : Inport
  __UniqueInportName__2__ : Inport  Port=2
  __UniqueInportName__3__ : Inport  Port=3
  __UniqueInportName__4__ : Inport  Port=4
  __UniqueInportName__5__ : Inport  Port=5
  __UniqueInportName__6__ : Inport  Port=6
  __UniqueInportName__7__ : Inport  Port=7
  __UniqueInportName__8__ : Inport  Port=8
  __UniqueInportName__9__ : Inport  Port=9
  __UniqueInportName__10__ : Inport  Port=10
  __UniqueInportName__11__ : Inport  Port=11
  __UniqueInportName__12__ : Inport  Port=12
  Mux1 : BusCreator  Inputs=12
  motor_out : Outport
  wires:
  __UniqueInportName__1__/1 -> Mux1/1  "Stator current is_a (A)"
  __UniqueInportName__2__/1 -> Mux1/2  "Stator current is_b (A)"
  __UniqueInportName__3__/1 -> Mux1/3  "Stator current is_c (A)"
  __UniqueInportName__4__/1 -> Mux1/4  "Stator back EMF e_a (V)"
  __UniqueInportName__5__/1 -> Mux1/5  "Stator back EMF e_b (V)"
  __UniqueInportName__6__/1 -> Mux1/6  "Stator back EMF e_cV)"
  __UniqueInportName__7__/1 -> Mux1/7  "Hall effect signal h_a"
  __UniqueInportName__8__/1 -> Mux1/8  "Hall effect signal h_b"
  __UniqueInportName__9__/1 -> Mux1/9  "Hall effect signal h_c"
  __UniqueInportName__10__/1 -> Mux1/10  "Rotor speed wm (rad/s)"
  __UniqueInportName__11__/1 -> Mux1/11  "Rotor angle thetam (rad)"
  __UniqueInportName__12__/1 -> Mux1/12  "Electromagnetic torque Te (N*m)"
  Mux1/1 -> motor_out/1

== system BLDCmotorControl_FOC_R2017b/BLDC_model_open/signal_log6 ==
  i_DC : Inport
  Terminator_1 : Terminator
  wires:
  i_DC/1 -> Terminator_1/1  "i_DC"

== system BLDCmotorControl_FOC_R2017b/PWM_gates/PWM_generator1 ==
  DC : Inport  SampleTime=Ts
  PWM_generator_sfcn : S-Function  FunctionName=PWM_generator_sf  SFunctionModules=""  SFunctionDeploymentMode=off  EnableBusSupport=off  SFcnStateName=DWORK0  mask{rtw_sf_name=PWM_generator_sf, showVar=off}
      mask prompts: rtw_sf_name "Simulink:masks:GenSFuncName_MP"; showVar "Simulink:masks:GenSFuncShowModuleList_MP"
      mask help: Simulink:masks:GenSFuncDesc_MD
      mask init: same as BLDCmotorControl_FOC_R2017b/BLDC_model_closed/BLDC_model_sfcn
      settings: SFcnIsStateOwnerBlock=on
      settings: CopyFcn=|
      | if ~strcmp(get_param(gcb,'Linkstatus'),'none') && ...
      | ~strcmp(get_param(gcb,'Linkstatus'),'implicit')
      |   set_param(gcb,'LinkStatus','none');
      | end
      mask Help: eval('feval(''rtwprivate'',''rtwhelpview'',''rtw_sfcn_block'')');
      mask Display:
      | port_label('input',1,'DC');
      | port_label('output',1,'PWM');
  __InputSSForSFun__ : Subsystem
  __OutputSSForSFun__ : Subsystem
  PWM : Outport
  wires:
  __OutputSSForSFun__/1(PWM) -> PWM/1
  PWM_generator_sfcn/1 -> __OutputSSForSFun__/1(__UniqueInportName__1__)
  __InputSSForSFun__/1(__UniqueOutportName__1__) -> PWM_generator_sfcn/1
  DC/1 -> __InputSSForSFun__/1(DC)

== system BLDCmotorControl_FOC_R2017b/PWM_gates/PWM_generator12 ==
  DC : Inport  SampleTime=Ts
  PWM_generator_sfcn : S-Function  FunctionName=PWM_generator_sf  SFunctionModules=""  SFunctionDeploymentMode=off  EnableBusSupport=off  SFcnStateName=DWORK0  mask{rtw_sf_name=PWM_generator_sf, showVar=off}
      mask prompts: rtw_sf_name "Simulink:masks:GenSFuncName_MP"; showVar "Simulink:masks:GenSFuncShowModuleList_MP"
      mask help: Simulink:masks:GenSFuncDesc_MD
      mask init: same as BLDCmotorControl_FOC_R2017b/BLDC_model_closed/BLDC_model_sfcn
      settings: SFcnIsStateOwnerBlock=on
      settings: CopyFcn=|
      | if ~strcmp(get_param(gcb,'Linkstatus'),'none') && ...
      | ~strcmp(get_param(gcb,'Linkstatus'),'implicit')
      |   set_param(gcb,'LinkStatus','none');
      | end
      mask Help: eval('feval(''rtwprivate'',''rtwhelpview'',''rtw_sfcn_block'')');
      mask Display:
      | port_label('input',1,'DC');
      | port_label('output',1,'PWM');
  __InputSSForSFun__ : Subsystem
  __OutputSSForSFun__ : Subsystem
  PWM : Outport
  wires:
  DC/1 -> __InputSSForSFun__/1(DC)
  __InputSSForSFun__/1(__UniqueOutportName__1__) -> PWM_generator_sfcn/1
  PWM_generator_sfcn/1 -> __OutputSSForSFun__/1(__UniqueInportName__1__)
  __OutputSSForSFun__/1(PWM) -> PWM/1

== system BLDCmotorControl_FOC_R2017b/PWM_gates/PWM_generator2 ==
  DC : Inport  SampleTime=Ts
  PWM_generator_sfcn : S-Function  FunctionName=PWM_generator_sf  SFunctionModules=""  SFunctionDeploymentMode=off  EnableBusSupport=off  SFcnStateName=DWORK0  mask{rtw_sf_name=PWM_generator_sf, showVar=off}
      mask prompts: rtw_sf_name "Simulink:masks:GenSFuncName_MP"; showVar "Simulink:masks:GenSFuncShowModuleList_MP"
      mask help: Simulink:masks:GenSFuncDesc_MD
      mask init: same as BLDCmotorControl_FOC_R2017b/BLDC_model_closed/BLDC_model_sfcn
      settings: SFcnIsStateOwnerBlock=on
      settings: CopyFcn=|
      | if ~strcmp(get_param(gcb,'Linkstatus'),'none') && ...
      | ~strcmp(get_param(gcb,'Linkstatus'),'implicit')
      |   set_param(gcb,'LinkStatus','none');
      | end
      mask Help: eval('feval(''rtwprivate'',''rtwhelpview'',''rtw_sfcn_block'')');
      mask Display:
      | port_label('input',1,'DC');
      | port_label('output',1,'PWM');
  __InputSSForSFun__ : Subsystem
  __OutputSSForSFun__ : Subsystem
  PWM : Outport
  wires:
  DC/1 -> __InputSSForSFun__/1(DC)
  __InputSSForSFun__/1(__UniqueOutportName__1__) -> PWM_generator_sfcn/1
  PWM_generator_sfcn/1 -> __OutputSSForSFun__/1(__UniqueInportName__1__)
  __OutputSSForSFun__/1(PWM) -> PWM/1

== system BLDCmotorControl_FOC_R2017b/PWM_gates/PWM_generator3 ==
  DC : Inport  SampleTime=Ts
  PWM_generator_sfcn : S-Function  FunctionName=PWM_generator_sf  SFunctionModules=""  SFunctionDeploymentMode=off  EnableBusSupport=off  SFcnStateName=DWORK0  mask{rtw_sf_name=PWM_generator_sf, showVar=off}
      mask prompts: rtw_sf_name "Simulink:masks:GenSFuncName_MP"; showVar "Simulink:masks:GenSFuncShowModuleList_MP"
      mask help: Simulink:masks:GenSFuncDesc_MD
      mask init: same as BLDCmotorControl_FOC_R2017b/BLDC_model_closed/BLDC_model_sfcn
      settings: SFcnIsStateOwnerBlock=on
      settings: CopyFcn=|
      | if ~strcmp(get_param(gcb,'Linkstatus'),'none') && ...
      | ~strcmp(get_param(gcb,'Linkstatus'),'implicit')
      |   set_param(gcb,'LinkStatus','none');
      | end
      mask Help: eval('feval(''rtwprivate'',''rtwhelpview'',''rtw_sfcn_block'')');
      mask Display:
      | port_label('input',1,'DC');
      | port_label('output',1,'PWM');
  __InputSSForSFun__ : Subsystem
  __OutputSSForSFun__ : Subsystem
  PWM : Outport
  wires:
  __OutputSSForSFun__/1(PWM) -> PWM/1
  PWM_generator_sfcn/1 -> __OutputSSForSFun__/1(__UniqueInportName__1__)
  __InputSSForSFun__/1(__UniqueOutportName__1__) -> PWM_generator_sfcn/1
  DC/1 -> __InputSSForSFun__/1(DC)

== system BLDCmotorControl_FOC_R2017b/PWM_gates/PWM_generator4 ==
  DC : Inport  SampleTime=Ts
  PWM_generator_sfcn : S-Function  FunctionName=PWM_generator_sf  SFunctionModules=""  SFunctionDeploymentMode=off  EnableBusSupport=off  SFcnStateName=DWORK0  mask{rtw_sf_name=PWM_generator_sf, showVar=off}
      mask prompts: rtw_sf_name "Simulink:masks:GenSFuncName_MP"; showVar "Simulink:masks:GenSFuncShowModuleList_MP"
      mask help: Simulink:masks:GenSFuncDesc_MD
      mask init: same as BLDCmotorControl_FOC_R2017b/BLDC_model_closed/BLDC_model_sfcn
      settings: SFcnIsStateOwnerBlock=on
      settings: CopyFcn=|
      | if ~strcmp(get_param(gcb,'Linkstatus'),'none') && ...
      | ~strcmp(get_param(gcb,'Linkstatus'),'implicit')
      |   set_param(gcb,'LinkStatus','none');
      | end
      mask Help: eval('feval(''rtwprivate'',''rtwhelpview'',''rtw_sfcn_block'')');
      mask Display:
      | port_label('input',1,'DC');
      | port_label('output',1,'PWM');
  __InputSSForSFun__ : Subsystem
  __OutputSSForSFun__ : Subsystem
  PWM : Outport
  wires:
  DC/1 -> __InputSSForSFun__/1(DC)
  __InputSSForSFun__/1(__UniqueOutportName__1__) -> PWM_generator_sfcn/1
  PWM_generator_sfcn/1 -> __OutputSSForSFun__/1(__UniqueInportName__1__)
  __OutputSSForSFun__/1(PWM) -> PWM/1

== system BLDCmotorControl_FOC_R2017b/PWM_gates/PWM_generator5 ==
  DC : Inport  SampleTime=Ts
  PWM_generator_sfcn : S-Function  FunctionName=PWM_generator_sf  SFunctionModules=""  SFunctionDeploymentMode=off  EnableBusSupport=off  SFcnStateName=DWORK0  mask{rtw_sf_name=PWM_generator_sf, showVar=off}
      mask prompts: rtw_sf_name "Simulink:masks:GenSFuncName_MP"; showVar "Simulink:masks:GenSFuncShowModuleList_MP"
      mask help: Simulink:masks:GenSFuncDesc_MD
      mask init: same as BLDCmotorControl_FOC_R2017b/BLDC_model_closed/BLDC_model_sfcn
      settings: SFcnIsStateOwnerBlock=on
      settings: CopyFcn=|
      | if ~strcmp(get_param(gcb,'Linkstatus'),'none') && ...
      | ~strcmp(get_param(gcb,'Linkstatus'),'implicit')
      |   set_param(gcb,'LinkStatus','none');
      | end
      mask Help: eval('feval(''rtwprivate'',''rtwhelpview'',''rtw_sfcn_block'')');
      mask Display:
      | port_label('input',1,'DC');
      | port_label('output',1,'PWM');
  __InputSSForSFun__ : Subsystem
  __OutputSSForSFun__ : Subsystem
  PWM : Outport
  wires:
  __OutputSSForSFun__/1(PWM) -> PWM/1
  PWM_generator_sfcn/1 -> __OutputSSForSFun__/1(__UniqueInportName__1__)
  __InputSSForSFun__/1(__UniqueOutportName__1__) -> PWM_generator_sfcn/1
  DC/1 -> __InputSSForSFun__/1(DC)

== system BLDCmotorControl_FOC_R2017b/PWM_gates/signal_log6 ==
  PWM : Inport
  Terminator_1 : Terminator
  wires:
  PWM/1 -> Terminator_1/1  "PWM"

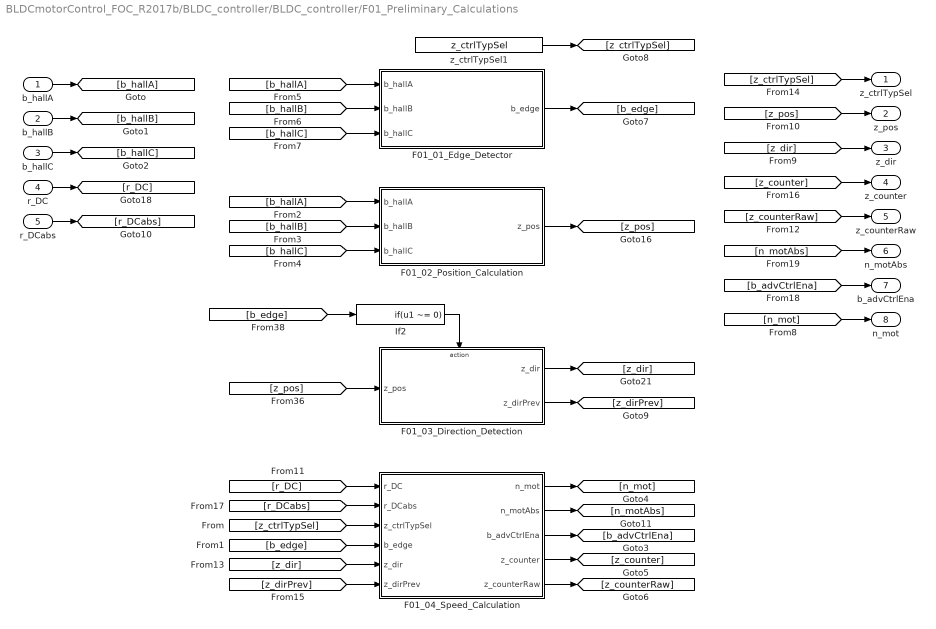
== system BLDCmotorControl_FOC_R2017b/BLDC_controller/BLDC_controller/F01_Preliminary_Calculations ==
  b_hallA : Inport
  b_hallB : Inport  Port=2
  b_hallC : Inport  Port=3
  r_DC : Inport  Port=4
  r_DCabs : Inport  Port=5
  F01_01_Edge_Detector : Subsystem
  F01_02_Position_Calculation : Subsystem
  F01_03_Direction_Detection : Subsystem
  F01_04_Speed_Calculation : Subsystem
  If2 : If  IfExpression=u1 ~= 0  ShowElse=off
  z_ctrlTypSel1 : Constant  Value=z_ctrlTypSel  OutDataTypeStr=uint8
  z_ctrlTypSel : Outport  OutputWhenDisabled=reset  InitialOutput=0
  z_pos : Outport  Port=2  OutputWhenDisabled=reset  InitialOutput=0
  z_dir : Outport  Port=3  OutputWhenDisabled=reset  InitialOutput=0
  z_counter : Outport  Port=4  OutputWhenDisabled=reset  InitialOutput=0
  z_counterRaw : Outport  Port=5  OutputWhenDisabled=reset  InitialOutput=0
  n_motAbs : Outport  Port=6  OutputWhenDisabled=reset  InitialOutput=0
  b_advCtrlEna : Outport  Port=7
  "n_mot " : Outport  Port=8  OutputWhenDisabled=reset  InitialOutput=0
  wires:
  If2/1 -> F01_03_Direction_Detection/Action
  [b_edge] -> If2/1
  [z_pos] -> F01_03_Direction_Detection/1(z_pos)
  [b_hallA] -> F01_01_Edge_Detector/1(b_hallA)
  F01_01_Edge_Detector/1("b_edge ") -> [b_edge]
  F01_03_Direction_Detection/1(z_dir) -> [z_dir]
  [b_hallB] -> F01_01_Edge_Detector/2(b_hallB)
  [b_hallC] -> F01_01_Edge_Detector/3(b_hallC)
  b_hallA/1 -> [b_hallA]
  b_hallB/1 -> [b_hallB]
  b_hallC/1 -> [b_hallC]
  [b_hallC] -> F01_02_Position_Calculation/3(b_hallC)
  [b_hallB] -> F01_02_Position_Calculation/2(b_hallB)
  [b_hallA] -> F01_02_Position_Calculation/1(b_hallA)
  F01_02_Position_Calculation/1("z_pos ") -> [z_pos]
  [b_edge] -> F01_04_Speed_Calculation/4(b_edge)
  F01_04_Speed_Calculation/1(n_mot) -> [n_mot]
  [n_mot] -> "n_mot "/1
  [z_dir] -> z_dir/1
  [z_pos] -> z_pos/1
  [z_dir] -> F01_04_Speed_Calculation/5(z_dir)
  [z_ctrlTypSel] -> z_ctrlTypSel/1
  z_ctrlTypSel1/1 -> [z_ctrlTypSel]
  r_DC/1 -> [r_DC]
  [z_ctrlTypSel] -> F01_04_Speed_Calculation/3(z_ctrlTypSel)
  [r_DC] -> F01_04_Speed_Calculation/1(r_DC)
  [b_advCtrlEna] -> b_advCtrlEna/1
  F01_04_Speed_Calculation/3(b_advCtrlEna) -> [b_advCtrlEna]
  [z_counter] -> z_counter/1
  [z_counterRaw] -> z_counterRaw/1
  F01_04_Speed_Calculation/4(z_counter) -> [z_counter]
  F01_04_Speed_Calculation/5(z_counterRaw) -> [z_counterRaw]
  F01_03_Direction_Detection/2(z_dirPrev) -> [z_dirPrev]
  [z_dirPrev] -> F01_04_Speed_Calculation/6(z_dirPrev)
  r_DCabs/1 -> [r_DCabs]
  [r_DCabs] -> F01_04_Speed_Calculation/2(r_DCabs)
  F01_04_Speed_Calculation/2(n_motAbs) -> [n_motAbs]
  [n_motAbs] -> n_motAbs/1
